simulink model "Sim_Forcing_003h_expe_infra_transz_lim"  (Simulink 7.4)
settings: Solver=FixedStepDiscrete  StartTime=0.0  StopTime=inf  FixedStep=0.004  RelTol=1e-3
undefined symbols (not defined in the file or in its folder): DiscIntNeverNeededParam
libraries: simulink x39, gt_rt_lib x22, xpcutilitieslib x4, xpclib x2, dspswit3 x1
(part 4 of 4)

== system Sim_Forcing_003h_expe_infra_transz_lim/Breaking_Control 20/07/15/Move_cabin/expe_phase/Rate Control Dynamics X/Second-Order Filter, zeta 0.8 ==
  u : Inport
  T : Inport  Port=2  OutDataType=fixdt(1, 16)  OutScaling=2^0
  4*zeta*pi : Gain  Gain=3.2*pi  ParameterDataType=fixdt(1, 16)  ParameterScaling=2^0  OutDataTypeMode=double  OutDataType=fixdt(1, 16)  OutScaling=2^0  OutDataTypeStr=double
  4*zeta*pi/T_transfer /s : DiscreteIntegrator  gainval=1  SampleTime=0.004  OutDataType=fixdt(1, 16)  OutScaling=2^0  ICPrevOutput=DiscIntNeverNeededParam  ICPrevScaledInput=DiscIntNeverNeededParam
  Divide : Product  Inputs=*/  OutDataType=fixdt(1, 16)  OutScaling=2^-10
  Divide1 : Product  Inputs=*/  OutDataType=fixdt(1, 16)  OutScaling=2^-10
  Sum1 : Sum  Inputs=|+-  OutDataType=fixdt(1, 16)  OutScaling=2^0
  Sum2 : Sum  Inputs=-+|  OutDataType=fixdt(1, 16)  OutScaling=2^0
  pi/(zeta*T_transfer)/s : DiscreteIntegrator  gainval=1  SampleTime=0.004  OutDataType=fixdt(1, 16)  OutScaling=2^0  ICPrevOutput=DiscIntNeverNeededParam  ICPrevScaledInput=DiscIntNeverNeededParam
  pi/zeta : Gain  Gain=pi/0.8  ParameterDataType=fixdt(1, 16)  ParameterScaling=2^0  OutDataType=fixdt(1, 16)  OutScaling=2^0
  x : Outport
  wires:
  Divide/1 -> 4*zeta*pi/1
  Divide1/1 -> pi/zeta/1
  pi/zeta/1 -> pi/(zeta*T_transfer)/s/1
  pi/(zeta*T_transfer)/s/1 -> Sum2/1, x/1
  4*zeta*pi/T_transfer /s/1 -> Divide1/1, Sum1/2
  Sum1/1 -> Divide/1
  4*zeta*pi/1 -> 4*zeta*pi/T_transfer /s/1
  T/1 -> [T]
  [T] -> Divide/2
  [T] -> Divide1/2
  Sum2/1 -> Sum1/1
  u/1 -> Sum2/2

== system Sim_Forcing_003h_expe_infra_transz_lim/Breaking_Control 20/07/15/Move_cabin/expe_phase/Rate Control Dynamics X/Smooth Displacement Second-Order Filter, zeta 0.8 ==
  Step IN Reset on  either : Inport
  T : Inport  Port=2  OutDataType=fixdt(1, 16)  OutScaling=2^0
  (zeta*T_transfer)/pi : Gain  Gain=0.8/pi  ParameterDataType=fixdt(1, 16)  ParameterScaling=2^0  OutDataType=fixdt(1, 16)  OutScaling=2^0
  4*zeta*pi : Gain  Gain=3.2*pi  ParameterDataType=fixdt(1, 16)  ParameterScaling=2^0  OutDataType=fixdt(1, 16)  OutScaling=2^0
  4*zeta*pi/T_transfer /s : DiscreteIntegrator  gainval=1  ExternalReset=either  InitialConditionSource=external  SampleTime=0.004  OutDataType=fixdt(1, 16)  OutScaling=2^0  ICPrevOutput=DiscIntNeverNeededParam  ICPrevScaledInput=DiscIntNeverNeededParam
  Discrete Derivative : simulink/Discrete/Discrete Derivative  SystemSampleTime=-1  gainval=1.0  ICPrevScaledInput=0.0  OutMin=[]  OutMax=[]  OutDataType=fixdt(1, 16)  OutScaling=2^-10  DoSatur=off
  Divide : Product  Inputs=*/  OutDataType=fixdt(1, 16)  OutScaling=2^-10
  Divide1 : Product  Inputs=*/  OutDataType=fixdt(1, 16)  OutScaling=2^-10
  For saving position  and velocity until after switchover : UnitDelay  SampleTime=-1
  Product : Product  OutDataType=fixdt(1, 16)  OutScaling=2^0  RndMeth=Zero
  Sum1 : Sum  Inputs=|+-  OutDataType=fixdt(1, 16)  OutScaling=2^0
  Sum2 : Sum  Inputs=-+|  OutDataType=fixdt(1, 16)  OutScaling=2^0
  pi/(zeta*T_transfer)/s : DiscreteIntegrator  gainval=1  ExternalReset=either  InitialConditionSource=external  SampleTime=0.004  OutDataType=fixdt(1, 16)  OutScaling=2^0  ICPrevOutput=DiscIntNeverNeededParam  ICPrevScaledInput=DiscIntNeverNeededParam
  pi/zeta : Gain  Gain=pi/0.8  ParameterDataType=fixdt(1, 16)  ParameterScaling=2^0  OutDataType=fixdt(1, 16)  OutScaling=2^0
  Out : Outport
  wires:
  Discrete Derivative/1 -> Product/2
  Product/1 -> (zeta*T_transfer)/pi/1
  Divide/1 -> 4*zeta*pi/1
  Divide1/1 -> pi/zeta/1
  pi/zeta/1 -> pi/(zeta*T_transfer)/s/1
  pi/(zeta*T_transfer)/s/1 -> Sum2/1, Out/1, For saving position  and velocity until after switchover/1
  4*zeta*pi/T_transfer /s/1 -> Divide1/1, Sum1/2
  Sum1/1 -> Divide/1
  4*zeta*pi/1 -> 4*zeta*pi/T_transfer /s/1
  T/1 -> [T]
  Step IN Reset on  either/1 -> [Step], Sum2/2
  [Step] -> 4*zeta*pi/T_transfer /s/2
  [Step] -> pi/(zeta*T_transfer)/s/2
  [T] -> Divide/2
  For saving position  and velocity until after switchover/1 -> Discrete Derivative/1, pi/(zeta*T_transfer)/s/3
  [T] -> Product/1
  (zeta*T_transfer)/pi/1 -> 4*zeta*pi/T_transfer /s/3
  [T] -> Divide1/2
  Sum2/1 -> Sum1/1

== system Sim_Forcing_003h_expe_infra_transz_lim/Breaking_Control 20/07/15/Move_cabin/expe_phase/Rate Control Dynamics Y/Second-Order Filter, zeta 0.8 ==
  u : Inport
  T : Inport  Port=2  OutDataType=fixdt(1, 16)  OutScaling=2^0
  4*zeta*pi : Gain  Gain=3.2*pi  ParameterDataType=fixdt(1, 16)  ParameterScaling=2^0  OutDataTypeMode=double  OutDataType=fixdt(1, 16)  OutScaling=2^0  OutDataTypeStr=double
  4*zeta*pi/T_transfer /s : DiscreteIntegrator  gainval=1  SampleTime=0.004  OutDataType=fixdt(1, 16)  OutScaling=2^0  ICPrevOutput=DiscIntNeverNeededParam  ICPrevScaledInput=DiscIntNeverNeededParam
  Divide : Product  Inputs=*/  OutDataType=fixdt(1, 16)  OutScaling=2^-10
  Divide1 : Product  Inputs=*/  OutDataType=fixdt(1, 16)  OutScaling=2^-10
  Sum1 : Sum  Inputs=|+-  OutDataType=fixdt(1, 16)  OutScaling=2^0
  Sum2 : Sum  Inputs=-+|  OutDataType=fixdt(1, 16)  OutScaling=2^0
  pi/(zeta*T_transfer)/s : DiscreteIntegrator  gainval=1  SampleTime=0.004  OutDataType=fixdt(1, 16)  OutScaling=2^0  ICPrevOutput=DiscIntNeverNeededParam  ICPrevScaledInput=DiscIntNeverNeededParam
  pi/zeta : Gain  Gain=pi/0.8  ParameterDataType=fixdt(1, 16)  ParameterScaling=2^0  OutDataType=fixdt(1, 16)  OutScaling=2^0
  x : Outport
  wires:
  Divide/1 -> 4*zeta*pi/1
  Divide1/1 -> pi/zeta/1
  pi/zeta/1 -> pi/(zeta*T_transfer)/s/1
  pi/(zeta*T_transfer)/s/1 -> Sum2/1, x/1
  4*zeta*pi/T_transfer /s/1 -> Divide1/1, Sum1/2
  Sum1/1 -> Divide/1
  4*zeta*pi/1 -> 4*zeta*pi/T_transfer /s/1
  T/1 -> [T]
  [T] -> Divide/2
  [T] -> Divide1/2
  Sum2/1 -> Sum1/1
  u/1 -> Sum2/2

== system Sim_Forcing_003h_expe_infra_transz_lim/Breaking_Control 20/07/15/Move_cabin/expe_phase/Rate Control Dynamics Y/Smooth Displacement Second-Order Filter, zeta 0.8 ==
  Step IN Reset on  either : Inport
  T : Inport  Port=2  OutDataType=fixdt(1, 16)  OutScaling=2^0
  (zeta*T_transfer)/pi : Gain  Gain=0.8/pi  ParameterDataType=fixdt(1, 16)  ParameterScaling=2^0  OutDataType=fixdt(1, 16)  OutScaling=2^0
  4*zeta*pi : Gain  Gain=3.2*pi  ParameterDataType=fixdt(1, 16)  ParameterScaling=2^0  OutDataType=fixdt(1, 16)  OutScaling=2^0
  4*zeta*pi/T_transfer /s : DiscreteIntegrator  gainval=1  ExternalReset=either  InitialConditionSource=external  SampleTime=0.004  OutDataType=fixdt(1, 16)  OutScaling=2^0  ICPrevOutput=DiscIntNeverNeededParam  ICPrevScaledInput=DiscIntNeverNeededParam
  Discrete Derivative : simulink/Discrete/Discrete Derivative  SystemSampleTime=-1  gainval=1.0  ICPrevScaledInput=0.0  OutMin=[]  OutMax=[]  OutDataType=fixdt(1, 16)  OutScaling=2^-10  DoSatur=off
  Divide : Product  Inputs=*/  OutDataType=fixdt(1, 16)  OutScaling=2^-10
  Divide1 : Product  Inputs=*/  OutDataType=fixdt(1, 16)  OutScaling=2^-10
  For saving position  and velocity until after switchover : UnitDelay  SampleTime=-1
  Product : Product  OutDataType=fixdt(1, 16)  OutScaling=2^0  RndMeth=Zero
  Sum1 : Sum  Inputs=|+-  OutDataType=fixdt(1, 16)  OutScaling=2^0
  Sum2 : Sum  Inputs=-+|  OutDataType=fixdt(1, 16)  OutScaling=2^0
  pi/(zeta*T_transfer)/s : DiscreteIntegrator  gainval=1  ExternalReset=either  InitialConditionSource=external  SampleTime=0.004  OutDataType=fixdt(1, 16)  OutScaling=2^0  ICPrevOutput=DiscIntNeverNeededParam  ICPrevScaledInput=DiscIntNeverNeededParam
  pi/zeta : Gain  Gain=pi/0.8  ParameterDataType=fixdt(1, 16)  ParameterScaling=2^0  OutDataType=fixdt(1, 16)  OutScaling=2^0
  Out : Outport
  wires:
  Discrete Derivative/1 -> Product/2
  Product/1 -> (zeta*T_transfer)/pi/1
  Divide/1 -> 4*zeta*pi/1
  Divide1/1 -> pi/zeta/1
  pi/zeta/1 -> pi/(zeta*T_transfer)/s/1
  pi/(zeta*T_transfer)/s/1 -> Sum2/1, Out/1, For saving position  and velocity until after switchover/1
  4*zeta*pi/T_transfer /s/1 -> Divide1/1, Sum1/2
  Sum1/1 -> Divide/1
  4*zeta*pi/1 -> 4*zeta*pi/T_transfer /s/1
  T/1 -> [T]
  Step IN Reset on  either/1 -> [Step], Sum2/2
  [Step] -> 4*zeta*pi/T_transfer /s/2
  [Step] -> pi/(zeta*T_transfer)/s/2
  [T] -> Divide/2
  For saving position  and velocity until after switchover/1 -> Discrete Derivative/1, pi/(zeta*T_transfer)/s/3
  [T] -> Product/1
  (zeta*T_transfer)/pi/1 -> 4*zeta*pi/T_transfer /s/3
  [T] -> Divide1/2
  Sum2/1 -> Sum1/1

== system Sim_Forcing_003h_expe_infra_transz_lim/Breaking_Control 20/07/15/Move_cabin/expe_phase/Rate Control Dynamics Z/Second-Order Filter, zeta 0.8 ==
  u : Inport
  T : Inport  Port=2  OutDataType=fixdt(1, 16)  OutScaling=2^0
  4*zeta*pi : Gain  Gain=3.2*pi  ParameterDataType=fixdt(1, 16)  ParameterScaling=2^0  OutDataTypeMode=double  OutDataType=fixdt(1, 16)  OutScaling=2^0  OutDataTypeStr=double
  4*zeta*pi/T_transfer /s : DiscreteIntegrator  gainval=1  SampleTime=0.004  OutDataType=fixdt(1, 16)  OutScaling=2^0  ICPrevOutput=DiscIntNeverNeededParam  ICPrevScaledInput=DiscIntNeverNeededParam
  Divide : Product  Inputs=*/  OutDataType=fixdt(1, 16)  OutScaling=2^-10
  Divide1 : Product  Inputs=*/  OutDataType=fixdt(1, 16)  OutScaling=2^-10
  Sum1 : Sum  Inputs=|+-  OutDataType=fixdt(1, 16)  OutScaling=2^0
  Sum2 : Sum  Inputs=-+|  OutDataType=fixdt(1, 16)  OutScaling=2^0
  pi/(zeta*T_transfer)/s : DiscreteIntegrator  gainval=1  SampleTime=0.004  OutDataType=fixdt(1, 16)  OutScaling=2^0  ICPrevOutput=DiscIntNeverNeededParam  ICPrevScaledInput=DiscIntNeverNeededParam
  pi/zeta : Gain  Gain=pi/0.8  ParameterDataType=fixdt(1, 16)  ParameterScaling=2^0  OutDataType=fixdt(1, 16)  OutScaling=2^0
  x : Outport
  wires:
  Divide/1 -> 4*zeta*pi/1
  Divide1/1 -> pi/zeta/1
  pi/zeta/1 -> pi/(zeta*T_transfer)/s/1
  pi/(zeta*T_transfer)/s/1 -> Sum2/1, x/1
  4*zeta*pi/T_transfer /s/1 -> Divide1/1, Sum1/2
  Sum1/1 -> Divide/1
  4*zeta*pi/1 -> 4*zeta*pi/T_transfer /s/1
  T/1 -> [T]
  [T] -> Divide/2
  [T] -> Divide1/2
  Sum2/1 -> Sum1/1
  u/1 -> Sum2/2

== system Sim_Forcing_003h_expe_infra_transz_lim/Breaking_Control 20/07/15/Move_cabin/expe_phase/Rate Control Dynamics Z/Smooth Displacement Second-Order Filter, zeta 0.8 ==
  Step IN Reset on  either : Inport
  T : Inport  Port=2  OutDataType=fixdt(1, 16)  OutScaling=2^0
  (zeta*T_transfer)/pi : Gain  Gain=0.8/pi  ParameterDataType=fixdt(1, 16)  ParameterScaling=2^0  OutDataType=fixdt(1, 16)  OutScaling=2^0
  4*zeta*pi : Gain  Gain=3.2*pi  ParameterDataType=fixdt(1, 16)  ParameterScaling=2^0  OutDataType=fixdt(1, 16)  OutScaling=2^0
  4*zeta*pi/T_transfer /s : DiscreteIntegrator  gainval=1  ExternalReset=either  InitialConditionSource=external  SampleTime=0.004  OutDataType=fixdt(1, 16)  OutScaling=2^0  ICPrevOutput=DiscIntNeverNeededParam  ICPrevScaledInput=DiscIntNeverNeededParam
  Discrete Derivative : simulink/Discrete/Discrete Derivative  SystemSampleTime=-1  gainval=1.0  ICPrevScaledInput=0.0  OutMin=[]  OutMax=[]  OutDataType=fixdt(1, 16)  OutScaling=2^-10  DoSatur=off
  Divide : Product  Inputs=*/  OutDataType=fixdt(1, 16)  OutScaling=2^-10
  Divide1 : Product  Inputs=*/  OutDataType=fixdt(1, 16)  OutScaling=2^-10
  For saving position  and velocity until after switchover : UnitDelay  SampleTime=-1
  Product : Product  OutDataType=fixdt(1, 16)  OutScaling=2^0  RndMeth=Zero
  Sum1 : Sum  Inputs=|+-  OutDataType=fixdt(1, 16)  OutScaling=2^0
  Sum2 : Sum  Inputs=-+|  OutDataType=fixdt(1, 16)  OutScaling=2^0
  pi/(zeta*T_transfer)/s : DiscreteIntegrator  gainval=1  ExternalReset=either  InitialConditionSource=external  SampleTime=0.004  OutDataType=fixdt(1, 16)  OutScaling=2^0  ICPrevOutput=DiscIntNeverNeededParam  ICPrevScaledInput=DiscIntNeverNeededParam
  pi/zeta : Gain  Gain=pi/0.8  ParameterDataType=fixdt(1, 16)  ParameterScaling=2^0  OutDataType=fixdt(1, 16)  OutScaling=2^0
  Out : Outport
  wires:
  Discrete Derivative/1 -> Product/2
  Product/1 -> (zeta*T_transfer)/pi/1
  Divide/1 -> 4*zeta*pi/1
  Divide1/1 -> pi/zeta/1
  pi/zeta/1 -> pi/(zeta*T_transfer)/s/1
  pi/(zeta*T_transfer)/s/1 -> Sum2/1, Out/1, For saving position  and velocity until after switchover/1
  4*zeta*pi/T_transfer /s/1 -> Divide1/1, Sum1/2
  Sum1/1 -> Divide/1
  4*zeta*pi/1 -> 4*zeta*pi/T_transfer /s/1
  T/1 -> [T]
  Step IN Reset on  either/1 -> [Step], Sum2/2
  [Step] -> 4*zeta*pi/T_transfer /s/2
  [Step] -> pi/(zeta*T_transfer)/s/2
  [T] -> Divide/2
  For saving position  and velocity until after switchover/1 -> Discrete Derivative/1, pi/(zeta*T_transfer)/s/3
  [T] -> Product/1
  (zeta*T_transfer)/pi/1 -> 4*zeta*pi/T_transfer /s/3
  [T] -> Divide1/2
  Sum2/1 -> Sum1/1

== matlab function Breaking_Control 20/07/15/Move UP1/add x_offset/Embedded MATLAB Function ==
  data: dx input double; set_out output double; set_in input double
function set_out = add_x_offset(dx, set_in)
%#eml

set_out = set_in;
set_out(3,1) = set_in(3,1) + dx;

== matlab function Breaking_Control 20/07/15/Timeline/Embedded MATLAB Function ==
  data: connect_x input double; u input double; y output double; flag_in input double; ac_in input double; ac_out output double
function [y,ac_out]  = fcn(connect_x,u,flag_in,ac_in)
%#eml
ac_out=ac_in;

if(u>0.01)
    ac_out=1;
    y=1;
else
if(ac_out==1)
    y=1;
    ac_out=1;
else
    y=0;
    ac_out=0;
end    
end

if(flag_in==1)
    ac_out=0;
    y=0;    
end

if(connect_x==0)
    y=0;  
	ac_out=0;
end

end

== matlab function Breaking_Control 20/07/15/Move_cabin/expe_phase/Stay within ellipse 20/07/15/Get R ==
  data: x input double; y input double; R output double
function R = fcn(x,y)
%#eml

R = sqrt(x*x+y*y);

== matlab function Breaking_Control 20/07/15/Timeline/Embedded MATLAB Function1 ==
  data: Tarest input double; stim_time input double; start_next output double
function start_next   = fcn(Tarest,stim_time)
%#eml

if(stim_time>=Tarest+5)
    start_next=1;
else 
    start_next=0;
end

end

== matlab function Breaking_Control 20/07/15/Move_cabin/expe_phase/Embedded MATLAB Function1 ==
  data: x input double; y output double; x_max input double; x_min input double; margin_max input double; margin_min input double; y_in input double; gain output double
function [y, gain] = final_soft_limit( x, x_max, x_min, margin_max, margin_min,y_in)

%--------------------------------------------------------------------------
%
%   argin_max and margin_min are the margins in which the exponetial
%   saturation takes place
%
%   x_max, x_min and margin_max and margin_min allow to compute the
%   factor between 0 and 1 of x_max and x_min of the linear range
%
%   Please note that x_max and x_min, margin_max and margin_min, are
%   all positive values; where the max is for the positive values of x and 
%   the min for the negative values
%
%--------------------------------------------------------------------------
   
    if x < x_max - margin_max && x >= 0
        y = x;
        gain=1;
    elseif x > -x_min + margin_min && x < 0
        y = x;
        gain=1;
    elseif x >= x_max - margin_max
        x1 = (x - x_max + margin_max);
        y = x_max*(1 -  margin_max/x_max*exp(-abs(x1)/margin_max));
        gain=exp(-abs(x1)/margin_max);

    else
        x1 = (x + x_min - margin_min);
        y = -x_min*(1 -  margin_min/x_min*exp(-abs(x1)/margin_min));
        gain=exp(-abs(x1)/margin_max);
    end
end

== matlab function Breaking_Control 20/07/15/Move_cabin/expe_phase/Embedded MATLAB Function2 ==
  data: x input double; y output double; x_max input double; x_min input double; margin_max input double; margin_min input double; y_in input double; gain output double
function [y,gain] = final_soft_limit( x, x_max, x_min, margin_max, margin_min,y_in)

%--------------------------------------------------------------------------
%
%   argin_max and margin_min are the margins in which the exponetial
%   saturation takes place
%
%   x_max, x_min and margin_max and margin_min allow to compute the
%   factor between 0 and 1 of x_max and x_min of the linear range
%
%   Please note that x_max and x_min, margin_max and margin_min, are
%   all positive values; where the max is for the positive values of x and 
%   the min for the negative values
%
%--------------------------------------------------------------------------
%    
%     if x < x_max - margin_max && x >= 0
%         y = x;
%     elseif x > -x_min + margin_min && x < 0
%         y = x;
%     elseif x >= x_max - margin_max
%         x1 = (x - x_max + margin_max);
%         y = x_max*(1 -  margin_max/x_max*exp(-abs(x1)/margin_max));
%     else
%         x1 = (x + x_min - margin_min);
%         y = -x_min*(1 -  margin_min/x_min*exp(-abs(x1)/margin_min));
%     end
    if x < x_max - margin_max && x >= 0
        y = x;
        gain=1;
    elseif x > -x_min + margin_min && x < 0
        y = x;
        gain=1;
    elseif x >= x_max - margin_max
        x1 = (x - x_max + margin_max);
        y = x_max*(1 -  margin_max/x_max*exp(-abs(x1)/margin_max));
        gain=exp(-abs(x1)/margin_max);

    else
        x1 = (x + x_min - margin_min);
        y = -x_min*(1 -  margin_min/x_min*exp(-abs(x1)/margin_min));
        gain=exp(-abs(x1)/margin_max);

    end

end

== matlab function Breaking_Control 20/07/15/Move_cabin/Subsystem/Embedded MATLAB Function3 ==
  data: com_or input double; max_tilt output double size=1
function max_tilt  = check_angle(com_or)
%#eml
max_tilt=max([abs(com_or(1)) abs(com_or(2)) abs(com_or(3))]);

    
end

== matlab function Breaking_Control 20/07/15/Move UP1/curve ==
  data: set input double; psi_set input double; x output double; fraction input double; z output double; psi output double; c output double; z_p output double
function [x, z, psi, c, z_p] = curve(set, psi_set, fraction)
%#eml
%**************************************************************************
%
% for fitting a parabolic curve through 3 points
%
%   set is a 3 x 2 matrix that include:
%       (x1, z1)
%       (x2, z2)
%       (x3, z3)
%
%   z is the abcis and x the ordinate of the curve
%   fraction runs from 0 to 1
%
%**************************************************************************

z_p = set(:,2);
x_p = set(:,1);

A = [z_p.*z_p z_p ones(3,1)];
c = A\x_p;

z = fraction*(z_p(3) - z_p(1)) + z_p(1);

x = [z.*z z 1]*c;

psi = fraction * psi_set;

== matlab function Breaking_Control 20/07/15/Move_cabin/expe_phase/Embedded MATLAB Function3 ==
  data: com_pos input double; T output double size=1; threshold input double
function T  = check_error(com_pos,threshold)
%#eml
%abs_yaw=abs(com_or(1))+abs(com_or(2))+abs(com_or(3))+abs(com_or(4));
max_tilt=max([abs(com_pos(1)) abs(com_pos(2)) abs(com_pos(3))]);

if(max_tilt>threshold)
    %T=max_tilt/2;
    T=max_tilt/3;
else
    T=7;%note: threshold should be 21
    %T=10; %note: threshold should be 20
    
end

== matlab function Joint Controller (May 7, 2015)1/Inverse Kinematics May 6, 2015/Simplified Inverse Kinematics/Simplified Inverse Kin/Embedded MATLAB Function2 ==
  data: vec input double; out output double
function out = MGDimose( vec )
out = zeros(6,1);

theta2=vec(2);
theta3=vec(3);
theta5=vec(5);

DTR=pi/180;
L1=0.5;
L2=1.3;
% L3=0.66;
% L4=0.365;
L5=0.29;
offset=0.055;
height_A2=1.045+1.06;
L34=1.025;%L3+L4;

cth23=cos(theta2*DTR+theta3*DTR);
sth23=sin(theta2*DTR+theta3*DTR);
cth2=cos(theta2*DTR);
sth2=sin(theta2*DTR);

theta = theta2+ theta3+ theta5;
X=100*(L2*cth2+L1+offset*sth23+L34*cth23+L5*cos(theta*DTR));
Z=-100*(L2*sth2+height_A2-offset*cth23+L34*sth23+L5*sin(theta*DTR));

out(1)=X;
out(3)=Z;
out(5)=theta;

== matlab function Joint Controller (May 7, 2015)1/Inverse Kinematics May 6, 2015/Simplified Inverse Kinematics/Simplified Inverse Kin/Embedded MATLAB Function3 ==
  data: vec input double; out output double
function out = MGIimose( vec )
out = zeros(7,1);

X=vec(1)/100;
Z=-vec(3)/100;
theta=vec(5);

theta2_in=vec(8);
theta3_in=vec(9);
theta5_in=vec(11);

DTR=pi/180;
% RTD=180/pi;

cth3i=cos(theta3_in*DTR);
sth3i=sin(theta3_in*DTR);
cth2i=cos(theta2_in*DTR);
cth23i=cos((theta2_in+theta3_in)*DTR);
sth23i=sin((theta2_in+theta3_in)*DTR);
% cth5i=cos(theta5_in*DTR);
% sth5i=sin(theta5_in*DTR);
cth=cos(theta);
sth=sin(theta);

 L1=0.5;
 L2=1.3;
% L3=0.66;
% L4=0.365;
 L5=0.29;
offset=0.055;
height_A2=1.045+1.06;
L34=1.025;%L3+L4;

%K=L2*L2+offset*offset+(L34)*(L34);
K=2.7437;

left_side= (((X-L1-L5*cth)*(X-L1-L5*cth)+(Z-height_A2-L5*sth)*(Z-height_A2-L5*sth)-K)/(2*L2))-(offset*cth+L34*sth)*sth3i-(-offset*sth+L34*cth)*cth3i;

%left_side=0.3325;

%equation to be solved:
% left_side= offset*sinus(theta3)+(L3+L4)cosinus(theta3)
%we assume theta3 is small
% syms theta3
% eqnth3 = left_side== offset*sin(theta3)+(L34)*cos(theta3);
% solth3=180*eval(solve(eqnth3,theta3))/pi;
% 
% for i=1:length(solth3)
%     if(solth3(i)<0)
%         theta3=solth3(i);
%     end
% end

dtheta3= left_side/((offset*cth+L34*sth)*cth3i-(-offset*sth+L34*cth)*sth3i);
if(abs(dtheta3)>0.01)
    dtheta3=sign(dtheta3)*0.01;
end
theta3=theta3_in+dtheta3;


% syms theta5
% alpha=L2*cos(theta3*pi/180)+(L34);
% beta=L2*sin(theta3*pi/180)+offset;
% eqnth5 = X-L1-L5 == alpha*cos(theta5)-beta*sin(theta5);
% solth5=180*eval(solve(eqnth5,theta5))/pi;
% 
% for i=1:length(solth5)
%     if(solth5(i)>0)
%         theta5=solth5(i);
%     end
% end

left_side_2=X-L1-L5*cth-L2*cth2i-offset*sth23i-L34*cth23i;

dtheta5= left_side_2/(offset*cth23i-L34*sth23i);
if(abs(dtheta5)>0.01)
    dtheta5=sign(dtheta5)*0.01;
end
theta5=theta5_in+dtheta5;

theta2=theta-theta3-theta5;

out(1)=0;
out(2)=theta2;
out(3)=theta3;
out(4)=0;
out(5)=theta5;
out(6)=0;

== matlab function Breaking_Control 20/07/15/compute_offset/Embedded MATLAB Function2 ==
  data: count input double; B parameter double; xytoz output double size=1; trigger input double; gradual_state output double; gs_in input double; xytoz_in input double; mod output double; current_axis output double
function [xytoz,gradual_state,mod,current_axis]   = check(count,B,trigger,gs_in,xytoz_in)
%#eml
current_axis=B(count,4);

if trigger==1
    if count==length(B)
        xytoz=xytoz_in;
        gradual_state=gs_in;
        
    else
        
        next_axis=B(count+1,4);
        
        if(current_axis==1||current_axis==2)
            if(next_axis==3)
                xytoz=1;
                gradual_state=1;
            else
                xytoz=0;
                gradual_state=0;
            end
        else
            if(next_axis==3)
                xytoz=1;
                gradual_state=1;
            else
                xytoz=0;
                gradual_state=0;
            end
        end
    end
    %mod=abs(gradual_state-1);
%     if(gradual_state==1)
%         mod=0;
%     else
%         if(current_axis==3)
%             mod=0;
%         else
%             mod=1;
%         end
%     end
else
    xytoz=xytoz_in;
    gradual_state=gs_in;
%     mod=abs(gradual_state-1);
%     if(gs_in==1)
%         mod=0;
%     else
%         mod=1;
%     end
end


if(gradual_state==1)
    mod=0;
else
    if(current_axis==3)
        mod=0;
    else
        mod=1;
    end
end



end

== matlab function Breaking_Control 20/07/15/compute_offset/Embedded MATLAB Function3 ==
  data: com_offset input double; status output double size=1; gradual_offset input double; threshold input double
function status  = check_progress(com_offset,gradual_offset,threshold)
%#eml
error=com_offset-gradual_offset;

max_error=max([abs(error(1)) abs(error(2))]);

if(max_error>threshold)
    status=0;
else
    status=1;
end

== matlab function Breaking_Control 20/07/15/Move_cabin/expe_phase/Embedded MATLAB Function5 ==
  data: x input double; y output double; x_max input double; x_min input double; margin_max input double; margin_min input double; y_in input double; gain output double
function [y,gain] = final_soft_limit( x, x_max, x_min, margin_max, margin_min,y_in)

%--------------------------------------------------------------------------
%
%   argin_max and margin_min are the margins in which the exponetial
%   saturation takes place
%
%   x_max, x_min and margin_max and margin_min allow to compute the
%   factor between 0 and 1 of x_max and x_min of the linear range
%
%   Please note that x_max and x_min, margin_max and margin_min, are
%   all positive values; where the max is for the positive values of x and 
%   the min for the negative values
%
%--------------------------------------------------------------------------
%    
%     if x < x_max - margin_max && x >= 0
%         y = x;
%     elseif x > -x_min + margin_min && x < 0
%         y = x;
%     elseif x >= x_max - margin_max
%         x1 = (x - x_max + margin_max);
%         y = x_max*(1 -  margin_max/x_max*exp(-abs(x1)/margin_max));
%     else
%         x1 = (x + x_min - margin_min);
%         y = -x_min*(1 -  margin_min/x_min*exp(-abs(x1)/margin_min));
%     end
    if x < x_max - margin_max && x >= 0
        y = x;
        gain=1;
    elseif x > -x_min + margin_min && x < 0
        y = x;
        gain=1;
    elseif x >= x_max - margin_max
        x1 = (x - x_max + margin_max);
        y = x_max*(1 -  margin_max/x_max*exp(-abs(x1)/margin_max));
        gain=exp(-abs(x1)/margin_max);

    else
        x1 = (x + x_min - margin_min);
        y = -x_min*(1 -  margin_min/x_min*exp(-abs(x1)/margin_min));
        gain=exp(-abs(x1)/margin_max);

    end

end

== matlab function Breaking_Control 20/07/15/select_ang_speed/Embedded MATLAB Function2 ==
  data: count input double; B parameter double; target_ang_speed output double size=3; endOffile_in input double; mask output double; vis_cond output double; flag_out output double; endOffile_out output double
function [target_ang_speed,mask,vis_cond,flag_out,endOffile_out]  = iterate(count,B,endOffile_in)
%#eml

mask=[0 0 0]';
flag_out=0;

if count>length(B)
endOffile_out=-1;
else endOffile_out=endOffile_in;
end

if endOffile_in<0 
    target_ang_speed=zeros(3,1);
    mask=[0 0 0]';
    vis_cond=1;
else target_ang_speed=B(count,1:3)';
    vis_cond=B(count,5);
    
%     if(target_ang_speed(1)~=0) 
%         mask(1)=1;
%     end
%     if(target_ang_speed(2)~=0) 
%         mask(2)=1;
%     end
%     if(target_ang_speed(3)~=0) 
%         mask(3)=1;
%         flag_out=-1;
%     end
    switch B(count,4)
        case 1
         mask=[1 0 0]';
         flag_out=0;
         case 2
         mask=[0 1 0]'; 
         flag_out=0;
        case 3
         mask=[0 0 1]';
         flag_out=-1;
    end


end

%%flag out is to take care that the next trial involves yaw and then a change in the starting position must be handled
if(B(count+1,4)==3)
    flag_out=1;
end

== matlab function Breaking_Control 20/07/15/Embedded MATLAB Function ==
  data: threshold input double; stick_out output double; enabled input double; stick_in input double
function stick_out = blank_zone(threshold,enabled,stick_in)
%#eml
stick_out=[0 0 0]';
if(enabled)

for i=1:3
    if(abs(stick_in(i))<threshold)
        stick_out(i)=0;
    else
        stick_out(i)=sign(stick_in(i))*(abs(stick_in(i))-threshold)/(1-threshold);
    end
end
else
stick_out =stick_in;  
end

== matlab function Joint Controller (May 7, 2015)1/Forward Kinematics/Embedded MATLAB Function ==
  data: vec input double; out output uint8
function out = ForKinSim( vec )
%--------------------------------------------------------------------------
%
%   This function solves the FORWARD kinematics of the 6-DOF KUKA arm and
%   wrist. This is the  version,
%   embedded in Simulink. The input and output are vectors that include the
%   list of parameters as defined herafter
%
%       *** Input variables, vec(1:13) ***
%
%   vec(1: 3)    POS         Room coordinates of flange, NED in cm
%   vec(4: 6)    EUL_ANG     Euler angles of the flange, phi, theta, psi, in deg
%   vec(1:6)     J_ANG_0     The joint angles, in deg
%
%       *** Output Variables ***
%
%   out(1: 3)    POS         Room coordinates of flange, NED in cm
%   out(4: 6)    EUL_ANG     Euler angles of the flange, phi, theta, psi, in deg
%
%   The North_East_Down convention is used and psi, theta, phi rotation
%   sequence; A2, A3, A5 are up positive and A4, A6 right rotation positive
%   Note that this is different from the KUKA convention
%
%   Written by Arthur J. Grunwald, Nov. 23, 2014
%
%--------------------------------------------------------------------------
%#eml

DTR = pi/180.;
RTD = 180/pi;

% reload variables
% the algorithm works in rad, so ang is in rad
J_ANG       = vec(1:6);   % Initial guess of the joint angles, in deg
ang         = J_ANG*DTR;

% reserve place for output
out = zeros(6,1);

% define length of arms
l1          = 50.;   % arm length in cm
l2          = 130.;
l3          = 66.;
l4          = 36.5;
l5          = 29.;
d           = 5.5;             % vertical offset of the center line of
% joint 4 from centerline of arm A3
Height_A2   = 104.5 + 106;     % height link A2 above the ground


% 4x4 Transfer matrices, include both rotation and translation

ang = adjust_ang( ang ); % ang is brought in the range +-pi
A1 = ang(1);
A2 = ang(2);
A3 = ang(3);
A4 = ang(4);
A5 = ang(5);
A6 = ang(6);

CA1 = cos(A1);
SA1 = sin(A1);
CA2 = cos(A2);
SA2 = sin(A2);
CA3 = cos(A3);
SA3 = sin(A3);
CA4 = cos(A4);
SA4 = sin(A4);
CA5 = cos(A5);
SA5 = sin(A5);
CA6 = cos(A6);
SA6 = sin(A6);

D1 = [CA1 -SA1 0 0; SA1 CA1 0 0; 0 0 1 0;  0 0 0 1];
D2 = [CA2 0 SA2 l1; 0 1 0 0; -SA2 0 CA2 0; 0 0 0 1];
D3 = [CA3 0 SA3 l2; 0 1 0 0; -SA3 0 CA3 0; 0 0 0 1];
D4 = [1 0 0 l3; 0 CA4 -SA4 0; 0 SA4 CA4 d; 0 0 0 1];
D5 = [CA5 0 SA5 l4; 0 1 0 0; -SA5 0 CA5 0; 0 0 0 1];
D6 = [1 0 0 l5; 0 CA6 -SA6 0; 0 SA6 CA6 0; 0 0 0 1];

% cut out the 3x3 DCM's for each of the transfer matrices
% Note that the DCM is for rotation from b->e
E1 = D1(1:3,1:3);
E2 = D2(1:3,1:3);
E3 = D3(1:3,1:3);
E4 = D4(1:3,1:3);
E5 = D5(1:3,1:3);
E6 = D6(1:3,1:3);

% --- computed position from links A1-A6 ---

x_cabin = [0; 0; 0];    % x,y,z cabin reference point (cm)
% to which the translation is made
x6 = [x_cabin; 1];
p = D1*D2*D3*D4*D5*D6*x6;
pos = p(1:3);        % position of the cabin reference point in the
% NED system (cm)

% computed Euler angles from links A1-A6
% Euler matrices for rotation from e->b (note the transpose)
E = E6'*E5'*E4'*E3'*E2'*E1';
eul_ang = DCM2Eul( E );

% place into output vector
out(1:3,1) = pos-[0;0;Height_A2];
out(4:6,1) = RTD*eul_ang;

end

== matlab function Joint Controller (May 7, 2015)1/Inverse Kinematics May 6, 2015/Inverse Kinematics/full inverse kin/Embedded MATLAB Function ==
  data: vec input double; out output double
function out = InvKinSim( vec )
%--------------------------------------------------------------------------
%
%   This function solves the inverse kinematics of the 6-DOF KUKA arm and
%   wrist by means of an iterative algorithm. This is the  version,
%   embedded in Simulink. The input and output are vectors that include the
%   list of parameters as defined herafter
%
%       *** Input variables, vec(1:13) ***
%
%   vec(1: 3)    POS         Room coordinates of flange, NED in cm
%   vec(4: 6)    EUL_ANG     Euler angles of the flange, phi, theta, psi, in deg
%   vec(7:12)    J_ANG_0     Initial guess of the joint angles, in deg
%
%       *** Output Variables ***
%
%   out(1:6)  J_ANG          The six joint angles after convergence
%   out(7)    N, error code  Number of iterations, when negative, it is an
%                            error code:
%                               -1 no convergence
%                               -2 out of reach of joints
%                               -3 joint angles exceeded
%
%   The North_East_Down convention is used and psi, theta, phi rotation
%   sequence; A2, A3, A5 are up positive and A4, A6 right rotation positive
%   Note that this is different from the KUKA convention
%
%   Written by Arthur J. Grunwald, Nov. 14, 2014
%   Re-written for Simulink embedded, Nov. 20, 2014
%
%--------------------------------------------------------------------------
%#eml
DTR = pi/180.;
RTD = 180/pi;

% reload variables
POS         = vec(1: 3);   % Room coordinates of flange, NED in cm
EUL_ANG     = vec(4: 6);   % Euler angles of the flange, phi, theta, psi, in deg
J_ANG_0     = vec(7:12);   % Initial guess of the joint angles, in deg
out         = zeros(7,1);  % reserve place for out

% soft limits on the links (NED convention)

% SL = [   175    130     88    200    61    200
%         -175    -20    -88   -200   -61   -200];

% Dec. 6, 2014: A2 and A3 limits changed to KUKA hardware
% May 7,2015 soft limits on the links (NED convention)
SL = [   159    129     87      349    60    349
        -159    -19    -87     -349   -60   -349];

% define length of arms
l1          = 50.;   % arm length in cm
l2          = 130.;
l3          = 66.;
l4          = 36.5;
l5          = 29.;
d           = 5.5;             % vertical offset of the center line of
% joint 4 from centerline of arm A3
Height_A2   = 104.5 + 106;     % height link A2 above the ground

% offset the height so that level zero is now at the height of the A2 joint
POS(3) = POS(3) + Height_A2;

% set initial guess; the algorithm works in rad, so ang is in rad
N = 0;
ang = J_ANG_0*DTR;

% check for maximum range of arm links and exit with n = 2 when exceeded
L = l2 + l3 + l4 + l5;
R = sqrt(L^2 - POS(3)^2) + l1;
R1 = sqrt(POS(1)^2 + POS(2)^2);
if R1 > R-5;
    out(1:6,1) = J_ANG_0; % return vector as is
    out(7,1)   = -2;
    return
end

%--------------------------------
% 	start of iterative loop
%--------------------------------

while(1)
    
    % 4x4 Transfer matrices, include both rotation and translation
    
    ang = adjust_ang( ang ); % ang is brought in the range +-pi
    A1 = ang(1);
    A2 = ang(2);
    A3 = ang(3);
    A4 = ang(4);
    A5 = ang(5);
    A6 = ang(6);
    
    CA1 = cos(A1);
    SA1 = sin(A1);
    CA2 = cos(A2);
    SA2 = sin(A2);
    CA3 = cos(A3);
    SA3 = sin(A3);
    CA4 = cos(A4);
    SA4 = sin(A4);
    CA5 = cos(A5);
    SA5 = sin(A5);
    CA6 = cos(A6);
    SA6 = sin(A6);
    
    D1 = [CA1 -SA1 0 0; SA1 CA1 0 0; 0 0 1 0;  0 0 0 1];
    D2 = [CA2 0 SA2 l1; 0 1 0 0; -SA2 0 CA2 0; 0 0 0 1];
    D3 = [CA3 0 SA3 l2; 0 1 0 0; -SA3 0 CA3 0; 0 0 0 1];
    D4 = [1 0 0 l3; 0 CA4 -SA4 0; 0 SA4 CA4 d; 0 0 0 1];
    D5 = [CA5 0 SA5 l4; 0 1 0 0; -SA5 0 CA5 0; 0 0 0 1];
    D6 = [1 0 0 l5; 0 CA6 -SA6 0; 0 SA6 CA6 0; 0 0 0 1];
    
    % cut out the 3x3 DCM's for each of the transfer matrices
    % Note that the DCM is for rotation from b->e
    E1 = D1(1:3,1:3);
    E2 = D2(1:3,1:3);
    E3 = D3(1:3,1:3);
    E4 = D4(1:3,1:3);
    E5 = D5(1:3,1:3);
    E6 = D6(1:3,1:3);
    
    % --- computed position from links A1-A6 ---
    
    %----------------------------------------------------------------------
    %   In order to move a point in the cabine in 6-DOF rather than the
    %   endplate, define the coordinates of that point in x_cabin
    %----------------------------------------------------------------------
    x_cabin = [0; 0; 0];    % x,y,z cabin reference point (cm)
    
    x6 = [x_cabin; 1];
    p = D1*D2*D3*D4*D5*D6*x6;
    pos = p(1:3);           % position of the cabin reference point in the
    % NED system (cm)
    
    % computed Euler angles from links A1-A6
    % Euler matrices for rotation from e->b (note the transpose)
    E = E6'*E5'*E4'*E3'*E2'*E1';
    eul_ang = DCM2Eul( E );
    
    % determine the vectors of rotation of the endplate in e-system
    % for each one of the links; this is a 3x6 matrix, when multiplied
    % with the vector of the joint angles, it will give the vector
    % of rotation of the endplate (and also of the cabin reference point)
    % in the NED system
    
    e6 = E1*E2*E3*E4*E5*[1 0 0]'; % x-axis
    e5 = E1*E2*E3*E4*   [0 1 0]'; % y-axis
    e4 = E1*E2*E3*      [1 0 0]'; % x-axis
    e3 = E1*E2*         [0 1 0]'; % y-axis
    e2 = E1*            [0 1 0]'; % y-axis
    e1 = eye(3)*        [0 0 1]'; % z-axis
    
    e = [e1 e2 e3 e4 e5 e6];
    
    % in order to see the changes in phi, theta, psi that this rotation
    % vector causes, we have to transform e->b first in yaw and after that
    % in pitch
    cs_psi = cos(eul_ang(3));
    sn_psi = sin(eul_ang(3));
    cs_tet = cos(eul_ang(2));
    sn_tet = sin(eul_ang(2));
    
    PSI = [cs_psi sn_psi 0; -sn_psi cs_psi 0; 0 0 1];
    TET = [cs_tet 0 -sn_tet; 0 1 0; sn_tet 0 cs_tet];
    e = TET*PSI*e;
    
    
    
    % the derivatives of D1-D6 for eah one of the link angles
    dD1 = [-SA1 -CA1 0 0; CA1 -SA1 0 0; 0 0 0 0; 0 0 0 0];
    dD2 = [-SA2 0 CA2 0; 0 0 0 0; -CA2 0 -SA2 0; 0 0 0 0];
    dD3 = [-SA3 0 CA3 0; 0 0 0 0; -CA3 0 -SA3 0; 0 0 0 0];
    dD4 = [0 0 0 0; 0 -SA4 -CA4 0; 0 CA4 -SA4 0; 0 0 0 0];
    dD5 = [-SA5 0 CA5 0; 0 0 0 0; -CA5 0 -SA5 0; 0 0 0 0];
    dD6 = [0 0 0 0; 0 -SA6 -CA6 0; 0 CA6 -SA6 0; 0 0 0 0];
    
    % Hessian Matrix H; the inverse of this matrix determines the link
    % angle speed as a function of the speed of x,y,z and the speed of the
    % Euler angles
    
    h1 = dD1*D2*D3*D4*D5*D6*x6;
    h2 = D1*dD2*D3*D4*D5*D6*x6;
    h3 = D1*D2*dD3*D4*D5*D6*x6;
    h4 = D1*D2*D3*dD4*D5*D6*x6;
    h5 = D1*D2*D3*D4*dD5*D6*x6;
    h6 = D1*D2*D3*D4*D5*dD6*x6;
    
    h = [h1 h2 h3 h4 h5 h6]; % this 3x6 is th upper half of H
    H = [h(1:3,:); e];       % the lower 3x6 half is the matrix e
    
    d_ang = inv(H) * [( POS - pos ); (DTR*EUL_ANG - eul_ang)];
    ang = ang + d_ang;
    ang = adjust_ang( ang );
    if(norm(d_ang) < 1.e-6)
        J_ANG = RTD*adjust_ang( ang );
        out(1:6,1) = J_ANG;
        out(7,1)   = N;
        break;
    end
    N = N + 1;
    
    % if more than 10 iterations, no convergence
    if N > 10
        out(1:6) = J_ANG_0; % return vector as is
        out(7)   = -1;
        return;
    end
end

% tests whether the links are within the set soft limits
for i = 1 : 6
    if J_ANG(i) >= SL(1,i)
        out(7,1) = -3;
        return;
    elseif J_ANG(i) <= SL(2,i)
        out(7,1) = -3;
        return;
    end
end

end

== matlab function Joint Controller (May 7, 2015)1/Inverse Kinematics May 6, 2015/Simplified Inverse Kinematics/Simplified Inverse Kin/Embedded MATLAB Function1 ==
  data: vec input double; out output double
function out = SimpleInvKin( vec )

% We use the NED convention
% This algorithm has a closed form solution and is based on the cosine rule
% However, due to the offset of the centerline of link A4 55 mm below the
% center of rotation of link A3, some small corrections have to be made;
% this is done iteratively by means of a second-order scheme.
% The gist of this routine is to show tha identical results are obtained
% with the fully-fledged 6-DOF inverse algorithm.
%
% The algorithm is also used for computing an initial guess for the
% fully-fledged inverse kinematics algorithm
% The initial guess uses only links A1, A2, A3 and assumes that the
% cabin at the end is straight and level and aligned with the arm
% Thus A4 and A6 are zero and A5 is A2 + A3
%
%   out(7) includes the parameter N
%       N > 0           the number of iterations needed to converge
%       N = -1          the iterative algorithm does not converge
%       N = -2          out of reachable limits
%       N -10<N<-30     upper limit of one of the joints A1-A6 exceeded
%       N -100<N<-110   upper limit of one of the joints A1-A6 exceeded
%
%   Written by Arthur Grunwald, November 11, 2014
%   Added correction because of offset of link A4, Dec 2, 2014
%   Added theta degree-of-freedom April 14, 2015
%   Modified the iterative scheme to second order NR scheme April 24, 2015
%   Modified FAR and CLOSE checks with intersecting circles May 6, 2015

RTD = 180/pi;
DTR = pi/180;

% May 7,2015 soft limits on the links (NED convention)
SL = [   159    129     87      349    60    349
        -159    -19    -87     -349   -60   -349];

% define length of the links

l1          = 50.;   % arm length in cm
l2          = 130.;
l3          = 66.;
l4          = 36.5;
l5          = 29.;
offset      = 5.5;             % vertical offset of the center line of
% joint 4 from centerline of arm A3
% joint 4 from centerline of arm A3
Height_A2   = 104.5 + 106;     % height link A2 above the ground

x = vec(1);
y = vec(2);
z = vec(3);

theta = vec(5);
cos_theta = cos(DTR*vec(5));
sin_theta = sin(DTR*vec(5));

N = 1;
out = zeros(7,1);

% compute dimensions of triangle
l = sqrt(x*x + y*y);
e = l - l1 - l5*cos_theta;
h = -(Height_A2 + z)-l5*sin_theta;
d = sqrt(e^2 + h^2);

% check whether the FAR location of C is reachable
b = l2;
c = l3 + l4;
margin = 5; % margin is 5 cm
if d > b + c - margin
    out(1:6,1) = vec(7:12); % return angles 'as is'
    out(3,1) = -90;
    out(7,1) = -2;
    return
end

% check whether the CLOSE location of C is reachable
if d + c - margin < b
    out(1:6,1) = vec(7:12); % return angles 'as is'
    out(3,1) = -90;
    out(7,1) = -2;
    return
end

% This iterative loop serves to correct for the offset of link A4
% A first good guess is to assume that beta is initially 90 deg
% A second-order scheme is used

A3 = vec(9);
beta = A3 + 180.;

while(1)
    
    sin_beta = sin(beta*DTR);
    sin2_beta = sin_beta*sin_beta;
    cos_beta = cos(beta*DTR);
    
    b = l2 - offset/sin_beta;
    c = l3 + l4 - offset*cos_beta/sin_beta;
    
    db_dbeta = offset * cos_beta/sin2_beta;
    dc_dbeta = offset/sin2_beta;
    
    A = (b*b + c*c - d*d);
    B = (2*b*c);
    dA_dbeta = (2*b*db_dbeta + 2*c*dc_dbeta);
    dB_dbeta = 2*(db_dbeta*c + b*dc_dbeta);
    eps = cos_beta - A/B;
    deps_dbeta = -sin_beta - (dA_dbeta*B - A*dB_dbeta)/B^2;
    dbeta = -RTD*eps/deps_dbeta;
    beta = beta + dbeta;
    
    if abs(dbeta) < 1.e-5
        break
    end
    N = N + 1;
    if N > 100
        N = -2;
        out(1:6,1) = vec(7:12); % return angles 'as is'
        out(3,1) = -90;
        out(7,1) = N;
        break;
    end
end

% employ cosine rule on angles alpha and beta of triangle
cos_alpha = (b*b + d*d - c*c)/(2*b*d);

alpha = RTD*acos(cos_alpha);
delta = RTD*atan2(h, e);

% the link angles
A1 = RTD*atan2(y, x);
A2 = alpha + delta;
A3 = beta - 180;
A4 = 0;
A5 = -(A2 + A3) + theta;
A6 = 0;

J_ANG = [A1 A2 A3 A4 A5 A6]';
out(1:6,1) = J_ANG;

% tests whether the links are within the set soft limits
for i = 1 : 6
    if J_ANG(i) >= SL(1,i)
        N = -10-i;
    elseif J_ANG(i) <= SL(2,i)
        N = -100-i;
    end
end

out(7,1) = N;

end
